simulink subsystem "coolantTemp"  (R2022b)
settings: Solver=VariableStepAuto  StartTime=0.0  StopTime=10.0  RelTol=1e-3
libraries: coolant x2
settings Model: Creator=serga  LastModifiedBy=serga

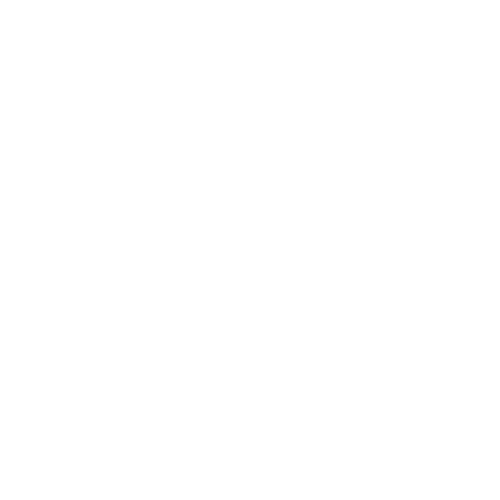
[thumbnail: Simulink's stored preview of the top-level diagram]
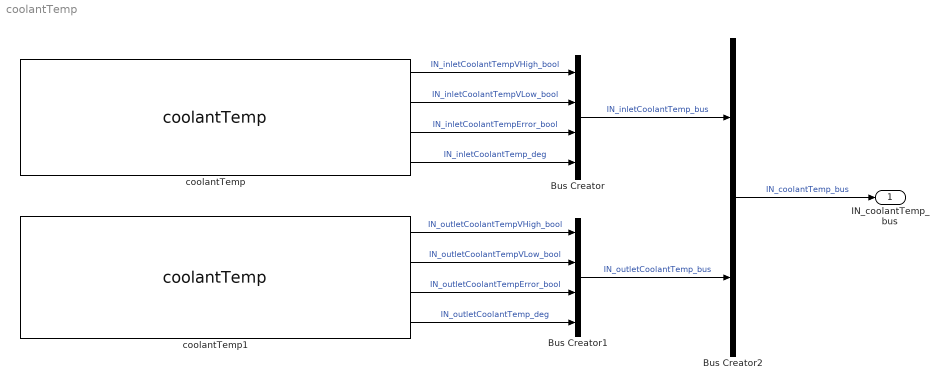
== system coolantTemp ==
  Bus Creator : BusCreator  Inputs=4
  Bus Creator1 : BusCreator  Inputs=4
  Bus Creator2 : BusCreator  Inputs=2
  coolantTemp : coolant/coolantTemp  pos='inlet'
      settings: LibrarySourceBlock=cooling/coolantTemp
  coolantTemp1 : coolant/coolantTemp  pos='outlet'
      settings: LibrarySourceBlock=cooling/coolantTemp
  IN_coolantTemp_bus : Outport
  wires:
  coolantTemp/1 -> Bus Creator/1  "IN_inletCoolantTempVHigh_bool"
  coolantTemp/2 -> Bus Creator/2  "IN_inletCoolantTempVLow_bool"
  coolantTemp/3 -> Bus Creator/3  "IN_inletCoolantTempError_bool"
  coolantTemp/4 -> Bus Creator/4  "IN_inletCoolantTemp_deg"
  coolantTemp1/1 -> Bus Creator1/1  "IN_outletCoolantTempVHigh_bool"
  coolantTemp1/2 -> Bus Creator1/2  "IN_outletCoolantTempVLow_bool"
  coolantTemp1/3 -> Bus Creator1/3  "IN_outletCoolantTempError_bool"
  coolantTemp1/4 -> Bus Creator1/4  "IN_outletCoolantTemp_deg"
  Bus Creator1/1 -> Bus Creator2/2  "IN_outletCoolantTemp_bus"
  Bus Creator/1 -> Bus Creator2/1  "IN_inletCoolantTemp_bus"
  Bus Creator2/1 -> IN_coolantTemp_bus/1  "IN_coolantTemp_bus"
